simulink model "TrabAzaurex"  (R2015a)
settings: Solver=ode45  StartTime=0.0  StopTime=10.0  RelTol=1e-3
libraries: powerlib x17
settings Model: Creator=Igor  LastModifiedBy=Igor

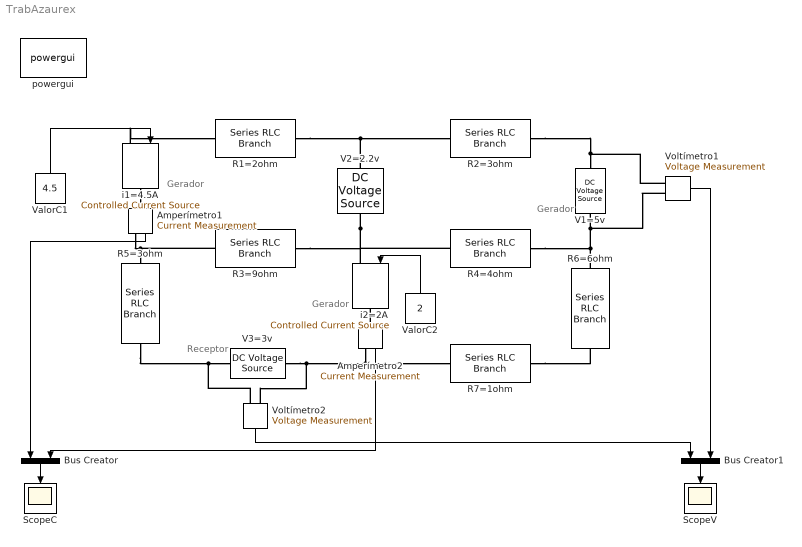
== system TrabAzaurex ==
  note: Gerador
  note: Receptor
  note: Gerador
  note: Gerador
  Amperímetro1 : powerlib/Measurements/Current Measurement  PhasorSimulation=off  OutputType=Complex  PSBequivalent=0
  Amperímetro2 : powerlib/Measurements/Current Measurement  PhasorSimulation=off  OutputType=Complex  PSBequivalent=0
  Bus Creator : BusCreator  Inputs=2
  Bus Creator1 : BusCreator  Inputs=2
  R1=2ohm : powerlib/Elements/Series RLC Branch  LConnTagsString=__new0  RConnTagsString=__new0  BranchType=R  Resistance=2  Inductance=1e-3  SetiL0=off  InitialCurrent=0  Capacitance=1e-6  Setx0=off  InitialVoltage=0  Measurements=None
  R2=3ohm : powerlib/Elements/Series RLC Branch  LConnTagsString=__new0  RConnTagsString=__new0  BranchType=R  Resistance=3  Inductance=1e-3  SetiL0=off  InitialCurrent=0  Capacitance=1e-6  Setx0=off  InitialVoltage=0  Measurements=None
  R3=9ohm : powerlib/Elements/Series RLC Branch  LConnTagsString=__new0  RConnTagsString=__new0  BranchType=R  Resistance=9  Inductance=1e-3  SetiL0=off  InitialCurrent=0  Capacitance=1e-6  Setx0=off  InitialVoltage=0  Measurements=None
  R4=4ohm : powerlib/Elements/Series RLC Branch  LConnTagsString=__new0  RConnTagsString=__new0  BranchType=R  Resistance=4  Inductance=1e-3  SetiL0=off  InitialCurrent=0  Capacitance=1e-6  Setx0=off  InitialVoltage=0  Measurements=None
  R5=3ohm : powerlib/Elements/Series RLC Branch  LConnTagsString=__new0  RConnTagsString=__new0  BranchType=R  Resistance=3  Inductance=1e-3  SetiL0=off  InitialCurrent=0  Capacitance=1e-6  Setx0=off  InitialVoltage=0  Measurements=None
  R6=6ohm : powerlib/Elements/Series RLC Branch  LConnTagsString=__new0  RConnTagsString=__new0  BranchType=R  Resistance=6  Inductance=1e-3  SetiL0=off  InitialCurrent=0  Capacitance=1e-6  Setx0=off  InitialVoltage=0  Measurements=None
  R7=1ohm : powerlib/Elements/Series RLC Branch  LConnTagsString=__new0  RConnTagsString=__new0  BranchType=R  Resistance=1  Inductance=1e-3  SetiL0=off  InitialCurrent=0  Capacitance=1e-6  Setx0=off  InitialVoltage=0  Measurements=None
  ScopeC : Scope
  ScopeV : Scope
      settings: SaveName=ScopeData3
  V1=5v : powerlib/Electrical Sources/DC Voltage Source  Amplitude=5  Measurements=Voltage
  V2=2.2v : powerlib/Electrical Sources/DC Voltage Source  Amplitude=2.2  Measurements=Voltage
  V3=3v : powerlib/Electrical Sources/DC Voltage Source  Amplitude=3  Measurements=Voltage
  ValorC1 : Constant  Value=4.5
  ValorC2 : Constant  Value=2
  Voltímetro1 : powerlib/Measurements/Voltage Measurement  PhasorSimulation=off  OutputType=Complex  PSBequivalent=0
  Voltímetro2 : powerlib/Measurements/Voltage Measurement  PhasorSimulation=off  OutputType=Complex  PSBequivalent=0
  i1=4.5A : powerlib/Electrical Sources/Controlled Current Source  Initialize=on  Source_Type=DC  Amplitude=4.5  Phase=0  Frequency=0  Measurements=Current
  "i2=2A " : powerlib/Electrical Sources/Controlled Current Source  Initialize=on  Source_Type=DC  Amplitude=2  Phase=0  Frequency=0  Measurements=Current
  powergui : powerlib/powergui  Priority=1  SimulationMode=Continuous  SolverType=Tustin/Backward Euler (TBE)  SampleTime=50e-6  frequency=60  SPID=off  DisableSnubberDevices=off  DisableRonSwitches=off  DisableVfSwitches=off  SwTol=0  DisplayEquations=off  Interpol=off  methode=off  Ts=100  FunctionMessages=off  echomessages=off  HookPort=off  EnableUseOfTLC=off  x0status=blocks  frequencyindice=0  Pbase=100e6  ErrMax=1e-4  Iterations=50  UnitsV=kV  UnitsW=MW  buscounter=0  RestoreLinks=warning  ResistiveCurrentMeasurement=off  Frange=[0:2:500]  Ylog=off  Xlog=on  ShowGrid=off  save=off  variable=ZData  structure=0  ZoomFFT=off  StartTime=0.0  cycles=1  DisplayStyle=1  fundamental=60  FreqAxis=off  MaxFrequency=1000  frequencyindicesteady=1  RmsSteady=1  display=off
  wires:
  Voltímetro2/1 -> Bus Creator1/1
  Voltímetro1/1 -> Bus Creator1/2
  Bus Creator1/1 -> ScopeV/1
  Bus Creator/1 -> ScopeC/1
  Amperímetro1/1 -> Bus Creator/1
  Amperímetro2/1 -> Bus Creator/2
  ValorC2/1 -> "i2=2A "/1
  ValorC1/1 -> i1=4.5A/1
  connections:
  R5=3ohm/RConn1 -- Voltímetro2/LConn2 -- V3=3v/RConn1
  V3=3v/LConn1 -- Voltímetro2/LConn1 -- Amperímetro2/RConn1 -- R7=1ohm/LConn1
  R7=1ohm/RConn1 -- R6=6ohm/RConn1
  R6=6ohm/LConn1 -- Voltímetro1/LConn2 -- V1=5v/LConn1 -- R4=4ohm/RConn1
  V2=2.2v/RConn1 -- "i2=2A "/LConn1 -- R4=4ohm/LConn1 -- R3=9ohm/RConn1
  R3=9ohm/LConn1 -- Amperímetro1/RConn1 -- R5=3ohm/LConn1
  R1=2ohm/RConn1 -- V2=2.2v/LConn1 -- R2=3ohm/LConn1
  R2=3ohm/RConn1 -- Voltímetro1/LConn1 -- V1=5v/RConn1
  Amperímetro2/LConn1 -- "i2=2A "/RConn1
  i1=4.5A/LConn1 -- R1=2ohm/LConn1
  i1=4.5A/RConn1 -- Amperímetro1/LConn1
